simulink model "compare_psk"  (R2022b)
settings: Solver=ode45  StartTime=0.0  StopTime=inf  RelTol=1e-3  EnableMultiTasking=on
values from neighbouring files (symbols this model uses):
  const = inphase + 1i*quadr    [signal.m]
  EbNodB = EbNoVec(n)    [compare_PSK_mod.m]
libraries: commdigbbndam3 x2, commchan3 x1, commsink2 x1, commrandsrc2 x1
settings Model: Creator=nazarova_a_a  LastModifiedBy=rando
settings SolverCC: AlgebraicLoopSolver=TrustRegion
settings DataIOCC: SaveFormat=Array  SignalLoggingSaveFormat=ModelDataLogs  SaveOutput=off  SaveTime=off  ReturnWorkspaceOutputs=off  SignalLoggingName=sigsOut
settings OptimizationCC: BlockReduction=off  BooleanDataType=off  ExpressionDepthLimit=2147483647  InitFltsAndDblsToZero=on  LifeSpan=inf
settings DebuggingCC: SaveWithParameterizedLinksMsg=none  UnderspecifiedInitializationDetection=Classic  MergeDetectMultiDrivingBlocksExec=none  SignalResolutionControl=TryResolveAllWithWarning  MultiTaskDSMMsg=warning  MultiTaskCondExecSysMsg=none  FcnCallInpInsideContextMsg=warning  UnconnectedInputMsg=warning  UnconnectedOutputMsg=warning  UnconnectedLineMsg=warning  StateNameClashWarn=warning  SFUnexpectedBacktrackingDiag=warning  SFNoUnconditionalDefaultTransitionDiag=warning  SFExecutionAtInitializationDiag=none  SFMachineParentedDataDiag=warning  ArithmeticOperatorsInVariantConditions=warning
settings HardwareCC: ProdBitPerPointer=32  ProdBitPerSizeT=32  ProdBitPerPtrDiffT=32  ProdLargestAtomicFloat=None  ProdIntDivRoundTo=Undefined  ProdEndianess=Unspecified  ProdWordSize=32  ProdHWDeviceType=32-bit Generic  TargetUnknown=on
settings ModelReferenceCC: PropagateSignalLabelsOutOfModel=off
settings SFSimCC: SimUseLocalCustomCode=off  CustomCodeUndefinedFunction=UseInterfaceOnly
settings RTWCC: RTWUseLocalCustomCode=off
settings CodeAppCC: StateflowObjectComments=on
settings GRTTargetCC: TargetFcnLib=ansi_tfl_tmw.mat  TargetLangStandard=C89/C90 (ANSI)  CombineOutputUpdateFcns=off  GRTInterface=on
settings ConfigComp: CovMetricSettings=dw  CovSaveCumulativeToWorkspaceVar=on  CovSaveSingleToWorkspaceVar=on

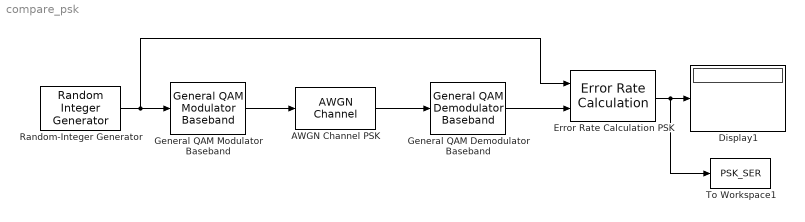
== system compare_psk ==
  AWGN Channel PSK : commchan3/AWGN Channel  InputProcessing=Columns as channels (frame based)  seed=1237  noiseMode="Signal to noise ratio  (Es/No)"  EbNodB=10  EsNodB=EbNodB+10*log10(6)  SNRdB=10  bitsPerSym=1  Ps=sum((abs(const)).^2)/length(const)  Tsym=1  variance=1
  Display1 : Display
  Error Rate Calculation PSK : commsink2/Error Rate Calculation  N=0  st_delay=0  cp_mode=Entire frame  subframe=[]  PMode=Port  WsName=ErrorVec  RsMode2=off  stop=on  numErr=1e4  maxBits=steps
  General QAM Demodulator Baseband : commdigbbndam3/General QAM Demodulator Baseband  SigCon=const  OutType=Integer  DecType=Hard decision  VarSource=Dialog  Variance=1  outDtypeBit=Inherit via internal rule  outDtype=Inherit via internal rule  roundingMode=Floor  overflowMode=Wrap  OvFlMode=off  OvFlModeLastStrValue=off  sigConstWordLen=16  sigConstDataTypeStr=Inherit: Same word length as input  sigConstLastDataTypeStr=Inherit: Same word length as input  accum1WordLen=32  accum1FracLen=30  prodInWordLen=32  prodInFracLen=30  prodInDataTypeStr=Inherit: Same as accumulator 1  prodInLastDataTypeStr=Inherit: Same as accumulator 1  prodOutWordLen=32  prodOutFracLen=30  accum2WordLen=32  accum2FracLen=30  accum3WordLen=32  accum3FracLen=30  nsiWordLen=32  nsiFracLen=30  nsiDataTypeStr=Inherit: Same as accumulator 3  nsiLastDataTypeStr=Inherit: Same as accumulator 3  invn0WordLen=16  invn0FracLen=8  invn0DataTypeStr=Inherit: Same word length as input  invn0LastDataTypeStr=Inherit: Same word length as input  outputWordLen=32  outputFracLen=30
  General QAM Modulator Baseband : commdigbbndam3/General QAM Modulator Baseband  SigCon=const  outDtype=double  outWordLen=16  outUDDataType=sfix(16)  outFracLenMode=Best precision  outFracLen=15  outDataTypeStr=double  outLastDataTypeStr=double
  Random-Integer Generator : commrandsrc2/Random Integer Generator  mul=length(const)  seed=12345  Ts=1  frameBased=on  sampPerFrame=10000  orient=off  outDataType=double
  To Workspace1 : ToWorkspace  VariableName=PSK_SER  SampleTime=-1
      settings: MaxDataPoints=1
  wires:
  AWGN Channel PSK/1 -> General QAM Demodulator Baseband/1
  General QAM Demodulator Baseband/1 -> Error Rate Calculation PSK/2
  Error Rate Calculation PSK/1 -> Display1/1, To Workspace1/1
  General QAM Modulator Baseband/1 -> AWGN Channel PSK/1
  Random-Integer Generator/1 -> Error Rate Calculation PSK/1, General QAM Modulator Baseband/1
